simulink model "RL_circuit"  (R2022b)
settings: Solver=VariableStepAuto  StartTime=0.0  StopTime=10.0  RelTol=1e-3
values from neighbouring files (symbols this model uses):
  airgap = [10 10.2070707071 10.4141414141 10.6212121212 10.8282828283 11.0353535354 11.2424242424 11.4494949495 11.6565656566 11.8636363636 12.0707070707 12.2777777778 ... (100 elements, 100x1)]    [force_airgap_current.mat]
  current = [-55 -53.8888888889 -52.7777777778 -51.6666666667 -50.5555555556 -49.4444444444 -48.3333333333 -47.2222222222 -46.1111111111 -45 -43.8888888889 -42.7777777778 ... (100 elements, 1x100)]    [force_airgap_current.mat]
undefined symbols (not defined in the file or in its folder): inductance, resistance, temperature
settings Model: Creator=USUARIO  LastModifiedBy=USUARIO

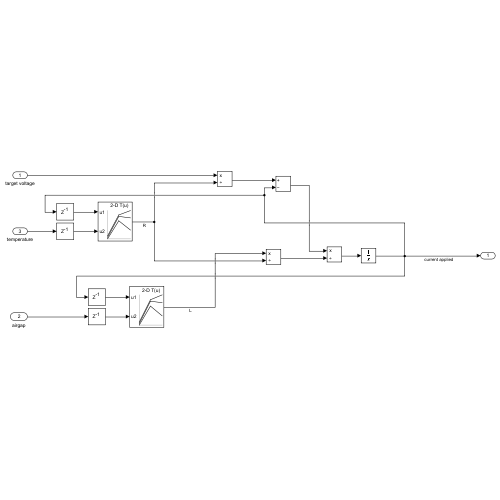
[thumbnail: Simulink's stored preview of the top-level diagram]
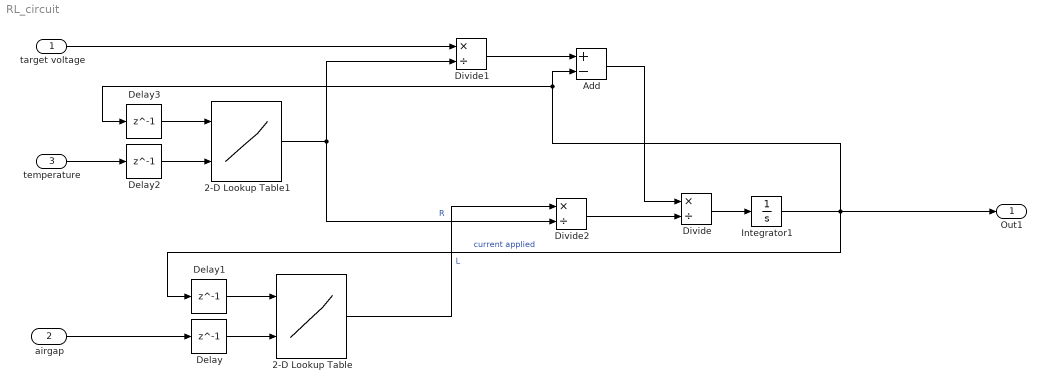
== system RL_circuit ==
  target voltage : Inport
  airgap : Inport  Port=2
  temperature : Inport  Port=3
  2-D Lookup Table : Lookup_n-D  BreakpointsForDimension1=current  BreakpointsForDimension2=airgap  Table=inductance  InternalRulePriority=Speed  RndMeth=Simplest
      settings: InputPortMap=u0,u1
  2-D Lookup Table1 : Lookup_n-D  BreakpointsForDimension1=current  BreakpointsForDimension2=temperature  Table=resistance  InternalRulePriority=Speed  RndMeth=Simplest
      settings: InputPortMap=u0,u1
  Add : Sum  Inputs=+-
  Delay{,1..3} (4 alike) : Delay  DelayLength=1
  Divide : Product  Inputs=*/
  Divide1 : Product  Inputs=*/
  Divide2 : Product  Inputs=*/
  Integrator1 : Integrator
  Out1 : Outport
  wires:
  2-D Lookup Table1/1 -> Divide2/2, Divide1/2  "R"
  Delay1/1 -> 2-D Lookup Table/1
  Divide2/1 -> Divide/2
  Divide1/1 -> Add/1
  2-D Lookup Table/1 -> Divide2/1  "L"
  Integrator1/1 -> Delay1/1, Out1/1, Delay3/1, Add/2  "current applied"
  Delay/1 -> 2-D Lookup Table/2
  Divide/1 -> Integrator1/1
  airgap/1 -> Delay/1
  Add/1 -> Divide/1
  Delay3/1 -> 2-D Lookup Table1/1
  temperature/1 -> Delay2/1
  Delay2/1 -> 2-D Lookup Table1/2
  target voltage/1 -> Divide1/1
